simulink model "Simulare_Model"  (R2023b)
settings: Solver=VariableStepAuto  StartTime=0.0  StopTime=10.0  RelTol=1e-3
values from neighbouring files (symbols this model uses):
  L = 4    [Params.m]
  T = 2    [Params.m]
settings Model: Creator=petri  LastModifiedBy=petri

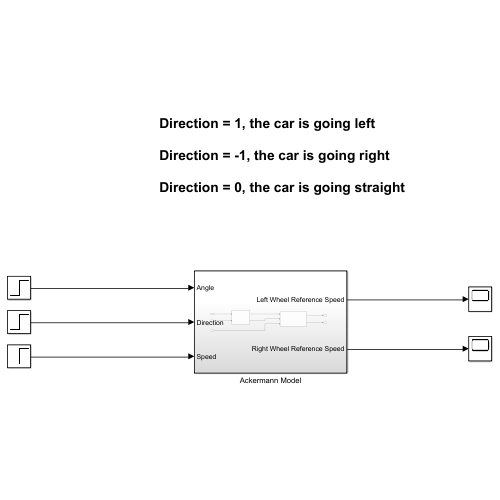
[thumbnail: Simulink's stored preview of the top-level diagram]
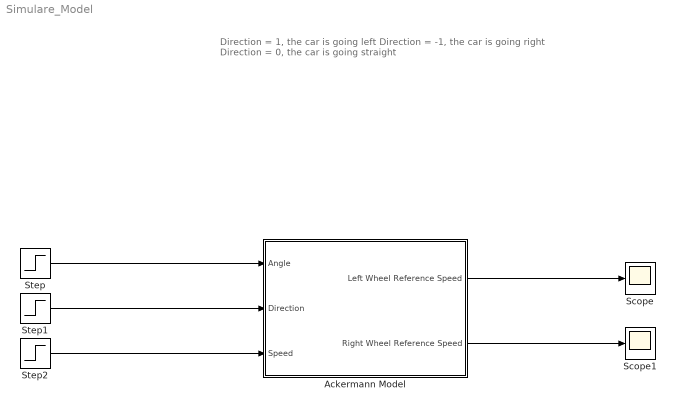
== system Simulare_Model ==
  note: Direction = 1, the car is going left
      |
      | Direction = -1, the car is going right
      |
      | Direction = 0, the car is going straight
  Ackermann Model : Subsystem
  Scope : Scope
  Scope1 : Scope
  Step : Step  Time=0  After=30  SampleTime=0
  Step1 : Step  Time=0  SampleTime=0
  Step2 : Step  Time=0  After=98  SampleTime=0
  wires:
  Step/1 -> Ackermann Model/1(Angle)
  Step1/1 -> Ackermann Model/2(Direction)
  Step2/1 -> Ackermann Model/3(Speed)
  Ackermann Model/1(Left Wheel Reference Speed) -> Scope/1
  Ackermann Model/2(Right Wheel Reference Speed) -> Scope1/1

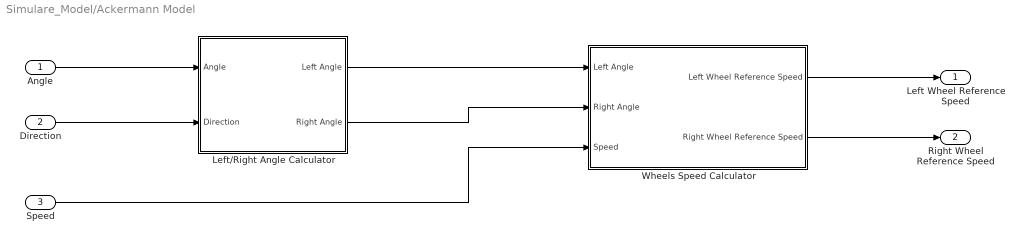
== system Simulare_Model/Ackermann Model ==
  Angle : Inport
  Direction : Inport  Port=2
  Speed : Inport  Port=3
  Left/Right Angle Calculator : Subsystem
  Wheels Speed Calculator : Subsystem
  Left Wheel Reference Speed : Outport
  Right Wheel Reference Speed : Outport  Port=2
  wires:
  Wheels Speed Calculator/1(Left Wheel Reference Speed) -> Left Wheel Reference Speed/1
  Left/Right Angle Calculator/2(Right Angle) -> Wheels Speed Calculator/2(Right Angle)
  Angle/1 -> Left/Right Angle Calculator/1(Angle)
  Left/Right Angle Calculator/1(Left Angle) -> Wheels Speed Calculator/1(Left Angle)
  Speed/1 -> Wheels Speed Calculator/3(Speed)
  Direction/1 -> Left/Right Angle Calculator/2(Direction)
  Wheels Speed Calculator/2(Right Wheel Reference Speed) -> Right Wheel Reference Speed/1

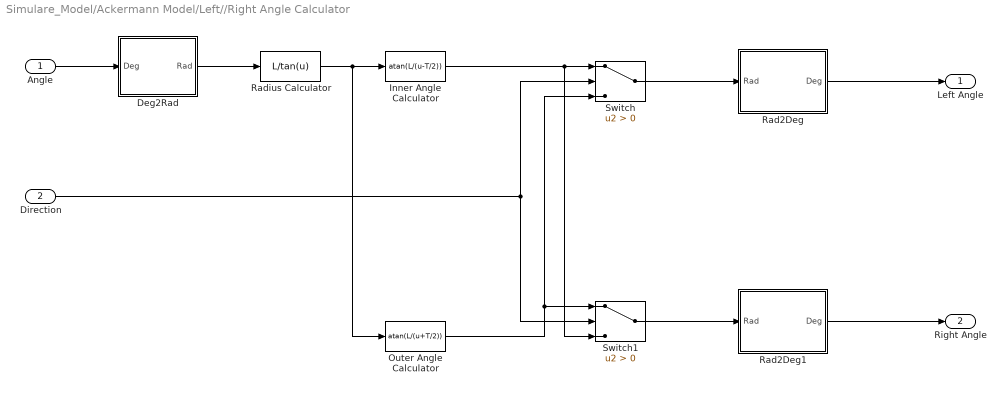
== system Simulare_Model/Ackermann Model/Left//Right Angle Calculator ==
  Angle : Inport
  Direction : Inport  Port=2
  Deg2Rad : Subsystem
  Inner Angle Calculator : Fcn  Expr=atan(L/(u-T/2))
  Outer Angle Calculator : Fcn  Expr=atan(L/(u+T/2))
  Rad2Deg : Subsystem
  Rad2Deg1 : Subsystem
  Radius Calculator : Fcn  Expr=L/tan(u)
  Switch : Switch  Criteria=u2 > Threshold  SaturateOnIntegerOverflow=off  InputSameDT=off
  Switch1 : Switch  Criteria=u2 > Threshold  SaturateOnIntegerOverflow=off  InputSameDT=off
  Left Angle : Outport
  Right Angle : Outport  Port=2
  wires:
  Direction/1 -> Switch/2, Switch1/2
  Angle/1 -> Deg2Rad/1(Deg)
  Outer Angle Calculator/1 -> Switch1/1, Switch/3
  Inner Angle Calculator/1 -> Switch/1, Switch1/3
  Switch/1 -> Rad2Deg/1(Rad)
  Switch1/1 -> Rad2Deg1/1(Rad)
  Rad2Deg1/1(Deg) -> Right Angle/1
  Rad2Deg/1(Deg) -> Left Angle/1
  Radius Calculator/1 -> Inner Angle Calculator/1, Outer Angle Calculator/1
  Deg2Rad/1(Rad) -> Radius Calculator/1

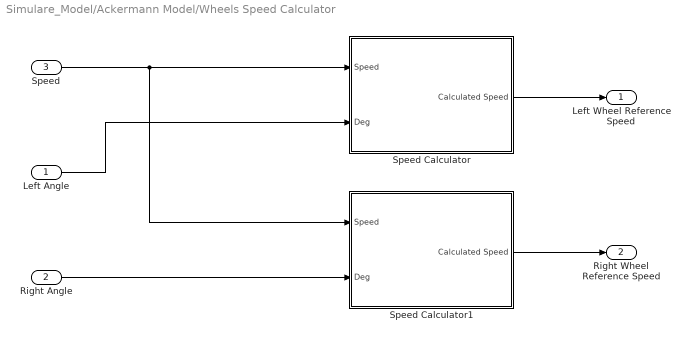
== system Simulare_Model/Ackermann Model/Wheels Speed Calculator ==
  Left Angle : Inport
  Right Angle : Inport  Port=2
  Speed : Inport  Port=3
  Speed Calculator : Subsystem
  Speed Calculator1 : Subsystem
  Left Wheel Reference Speed : Outport
  Right Wheel Reference Speed : Outport  Port=2
  wires:
  Speed Calculator1/1(Calculated Speed) -> Right Wheel Reference Speed/1
  Right Angle/1 -> Speed Calculator1/2(Deg)
  Speed/1 -> Speed Calculator/1(Speed), Speed Calculator1/1(Speed)
  Speed Calculator/1(Calculated Speed) -> Left Wheel Reference Speed/1
  Left Angle/1 -> Speed Calculator/2(Deg)

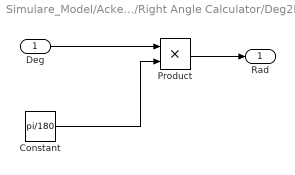
== system Simulare_Model/Ackermann Model/Left//Right Angle Calculator/Deg2Rad ==
  Deg : Inport
  Constant : Constant  Value=pi/180
  Product : Product
  Rad : Outport
  wires:
  Constant/1 -> Product/2
  Product/1 -> Rad/1
  Deg/1 -> Product/1

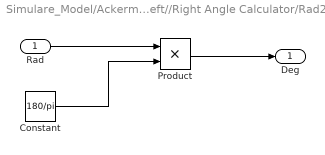
== system Simulare_Model/Ackermann Model/Left//Right Angle Calculator/Rad2Deg ==
  Rad : Inport
  Constant : Constant  Value=180/pi
  Product : Product
  Deg : Outport
  wires:
  Rad/1 -> Product/1
  Product/1 -> Deg/1
  Constant/1 -> Product/2

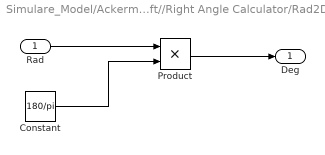
== system Simulare_Model/Ackermann Model/Left//Right Angle Calculator/Rad2Deg1 ==
  Rad : Inport
  Constant : Constant  Value=180/pi
  Product : Product
  Deg : Outport
  wires:
  Rad/1 -> Product/1
  Product/1 -> Deg/1
  Constant/1 -> Product/2

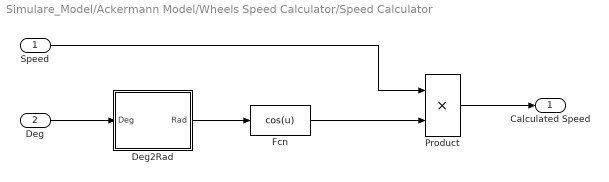
== system Simulare_Model/Ackermann Model/Wheels Speed Calculator/Speed Calculator ==
  Speed : Inport
  Deg : Inport  Port=2
  Deg2Rad : Subsystem
  Fcn : Fcn  Expr=cos(u)
  Product : Product
  Calculated Speed : Outport
  wires:
  Product/1 -> Calculated Speed/1
  Speed/1 -> Product/1
  Deg2Rad/1(Rad) -> Fcn/1
  Fcn/1 -> Product/2
  Deg/1 -> Deg2Rad/1(Deg)

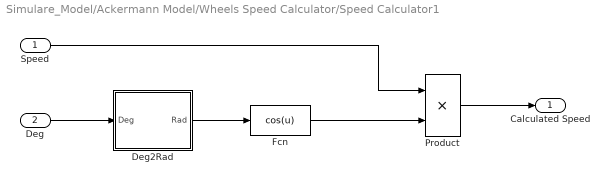
== system Simulare_Model/Ackermann Model/Wheels Speed Calculator/Speed Calculator1 ==
  Speed : Inport
  Deg : Inport  Port=2
  Deg2Rad : Subsystem
  Fcn : Fcn  Expr=cos(u)
  Product : Product
  Calculated Speed : Outport
  wires:
  Product/1 -> Calculated Speed/1
  Speed/1 -> Product/1
  Deg2Rad/1(Rad) -> Fcn/1
  Fcn/1 -> Product/2
  Deg/1 -> Deg2Rad/1(Deg)

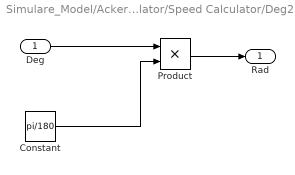
== system Simulare_Model/Ackermann Model/Wheels Speed Calculator/Speed Calculator/Deg2Rad ==
  Deg : Inport
  Constant : Constant  Value=pi/180
  Product : Product
  Rad : Outport
  wires:
  Constant/1 -> Product/2
  Product/1 -> Rad/1
  Deg/1 -> Product/1

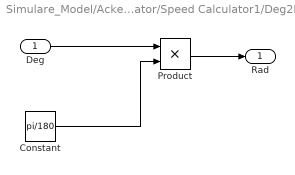
== system Simulare_Model/Ackermann Model/Wheels Speed Calculator/Speed Calculator1/Deg2Rad ==
  Deg : Inport
  Constant : Constant  Value=pi/180
  Product : Product
  Rad : Outport
  wires:
  Constant/1 -> Product/2
  Product/1 -> Rad/1
  Deg/1 -> Product/1
